simulink model "q3"  (Simulink 5.0)
settings: Solver=ode45  StartTime=0.0  StopTime=10.0  RelTol=1e-3
settings Model: LastModifiedBy=Thiago Araujo

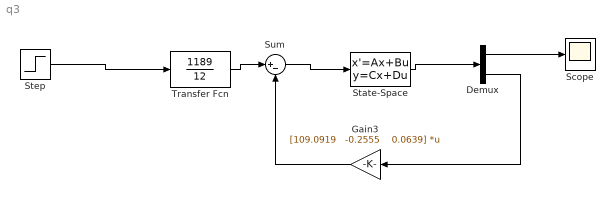
== system q3 ==
  Demux : Demux  Outputs=2
  Gain3 : Gain  Orientation=left  Gain="[109.0919   -0.2555    0.0639]"  Multiplication=Matrix(K*u) (u vector)  SaturateOnIntegerOverflow=on
  Scope : Scope
      settings: TimeRange=10  YMin=0  YMax=2e+047
  State-Space : StateSpace  A=[2 1 0; -5 -3.331e-016 1; 1196 1 -1]  B=[-4.337e-019; -2.082e-17; 1]  C=[10 21 4; 1 0 0; 0 1 0; 0 0 1]  D=[0; 0; 0; 0]
  Step : Step  Time=0  SampleTime=0
  Sum : Sum  Inputs=|+-  SaturateOnIntegerOverflow=on
  Transfer Fcn : TransferFcn  Numerator=[1189]  Denominator=[12]
  wires:
  Demux/1 -> Scope/1
  Demux/2 -> Gain3/1
  State-Space/1 -> Demux/1
  Gain3/1 -> Sum/2
  Sum/1 -> State-Space/1
  Transfer Fcn/1 -> Sum/1
  Step/1 -> Transfer Fcn/1
